simulink model "carro"  (R2015b)
settings: Solver=VariableStepAuto  StartTime=0.0  StopTime=50.0  RelTol=1e-3
values from neighbouring files (symbols this model uses):
  vo = vo_set(counter)    [Lab1.m]
  yo = 5    [Lab1.m]
undefined symbols (not defined in the file or in its folder): tau
settings Model: Creator=Alice  LastModifiedBy=Alice

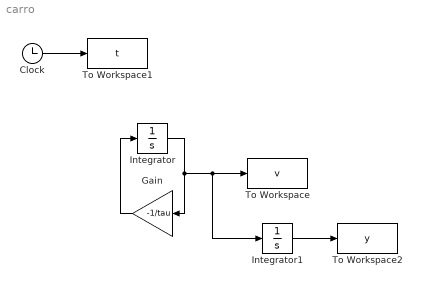
== system carro ==
  Clock : Clock
      settings: Decimation=tt
  Gain : Gain  Gain=-1/tau
  Integrator : Integrator  InitialCondition=vo
  Integrator1 : Integrator  InitialCondition=yo
  To Workspace : ToWorkspace  VariableName=v  SampleTime=-1
  To Workspace1 : ToWorkspace  VariableName=t  SampleTime=-1
  To Workspace2 : ToWorkspace  VariableName=y  SampleTime=-1
  wires:
  Integrator/1 -> Integrator1/1, To Workspace/1, Gain/1
  Gain/1 -> Integrator/1
  Clock/1 -> To Workspace1/1
  Integrator1/1 -> To Workspace2/1
